simulink model "HelicopterStateEstimation"  (R2023a)
settings: Solver=ode4  StartTime=0.0  StopTime=15  FixedStep=0.1  RelTol=1e-3
values from neighbouring files (symbols this model uses):
  A_c = [0, 0, 1, 0 ... (first row only)    [init.m]
  B_c = [0, 0 ... (first row only)    [init.m]
  B_p = 0.01    [init.m]
  B_y = 0.08    [init.m]
  C_c = [1,0,0,0 ... (first row only)    [init.m]
  g = 9.81    [init.m]
  j_eq_p = 0.0172    [init.m]
  j_eq_y = 0.0210    (= 0.021)    [init.m]
  K_pp = 0.0556    [init.m]
  K_py = 0.005    [init.m]
  K_yp = 0.15    [init.m]
  K_yy = 0.21084    [init.m]
  l_cm = 0.015    [init.m]
  m_heli = 0.479    [init.m]
  psi_op = pi/2    (= 1.57079632679)    [init.m]
  teta_op = -10*pi/180    (= -0.174532925199)    [init.m]
  V_mp_op = K_yy*m_heli*g*cos(teta_op)*l_cm/(K_yy*K_pp - K_yp*K_py)    [init.m]
  v_my_op = K_yp*V_mp_op/K_yy    [init.m]
  wpsi_op = 0    [init.m]
  wteta_op = 0    [init.m]
undefined symbols (not defined in the file or in its folder): L
libraries: simulink_extras x6
settings Model: Creator=Jardar Fagerlund  LastModifiedBy=Jardar Fagerlund

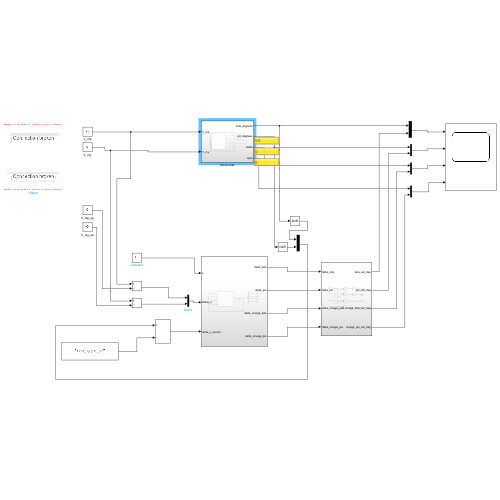
[thumbnail: Simulink's stored preview of the top-level diagram]
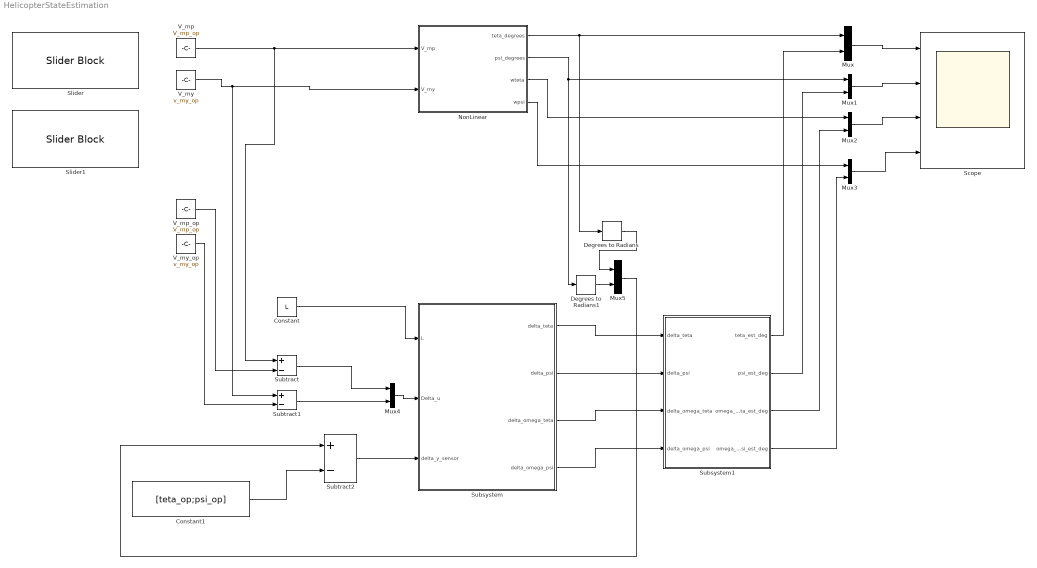
== system HelicopterStateEstimation ==
  Constant : Constant  Value=L
  Constant1 : Constant  Value=[teta_op;psi_op]
  Degrees to Radians : simulink_extras/Transformations/Degrees to Radians
  Degrees to Radians1 : simulink_extras/Transformations/Degrees to Radians
  Mux{,1..5} (6 alike) : Mux  Inputs=2
  NonLinear : Subsystem
  Scope : Scope  NumInputPorts=4
  Slider : SliderBlock  ScaleMin=1.1  ScaleMax=1.23
  Slider1 : SliderBlock  ScaleMin=0.4  ScaleMax=1
  Subsystem : Subsystem
  Subsystem1 : Subsystem
  Subtract : Sum  Inputs=+-
  Subtract1 : Sum  Inputs=+-
  Subtract2 : Sum  Inputs=+-
  V_mp : Constant  Value=V_mp_op
  V_mp_op : Constant  Value=V_mp_op
  V_my : Constant  Value=v_my_op
  V_my_op : Constant  Value=v_my_op
  wires:
  V_mp/1 -> Subtract/1, NonLinear/1(V_mp)
  V_my/1 -> NonLinear/2(V_my), Subtract1/1
  NonLinear/1(teta_degrees) -> Degrees to Radians/1, Mux/1
  NonLinear/2(psi_degrees) -> Degrees to Radians1/1, Mux1/1
  Mux/1 -> Scope/1
  Mux1/1 -> Scope/2
  Mux2/1 -> Scope/3
  Mux3/1 -> Scope/4
  NonLinear/3(wteta) -> Mux2/1
  NonLinear/4(wpsi) -> Mux3/1
  V_my_op/1 -> Subtract1/2
  Constant/1 -> Subsystem/1(L)
  Subtract/1 -> Mux4/1
  Subtract1/1 -> Mux4/2
  Mux4/1 -> Subsystem/2(Delta_u)
  Subtract2/1 -> Subsystem/3(delta_y_sensor)
  Constant1/1 -> Subtract2/2
  Mux5/1 -> Subtract2/1
  V_mp_op/1 -> Subtract/2
  Subsystem/1(delta_teta) -> Subsystem1/1(delta_teta)
  Subsystem/2(delta_psi) -> Subsystem1/2(delta_psi)
  Subsystem/3(delta_omega_teta) -> Subsystem1/3(delta_omega_teta)
  Subsystem/4(delta_omega_psi) -> Subsystem1/4(delta_omega_psi)
  Subsystem1/1(teta_est_deg) -> Mux/2
  Subsystem1/2(psi_est_deg) -> Mux1/2
  Subsystem1/3(omega_teta_est_deg) -> Mux2/2
  Subsystem1/4(omega_psi_est_deg) -> Mux3/2
  Degrees to Radians1/1 -> Mux5/2
  Degrees to Radians/1 -> Mux5/1

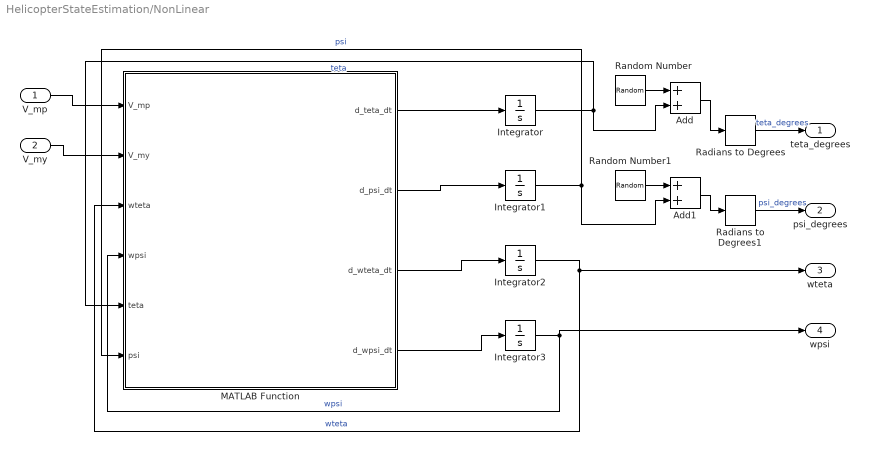
== system HelicopterStateEstimation/NonLinear ==
  V_mp : Inport
  V_my : Inport  Port=2
  Add : Sum
  Add1 : Sum
  Integrator : Integrator  InitialCondition=teta_op  LimitOutput=on  UpperSaturationLimit=35*pi/180  LowerSaturationLimit=-45*pi/180
  Integrator1 : Integrator  InitialCondition=psi_op  LimitOutput=on  UpperSaturationLimit=pi  LowerSaturationLimit=0
  Integrator2 : Integrator  InitialCondition=wteta_op
  Integrator3 : Integrator  InitialCondition=wpsi_op
  MATLAB Function : MATLAB Function  TreatAsAtomicUnit=on
  Radians to Degrees : simulink_extras/Transformations/Radians to Degrees
  Radians to Degrees1 : simulink_extras/Transformations/Radians to Degrees
  Random Number : RandomNumber  Variance=0.01
  Random Number1 : RandomNumber  Variance=0.01
  teta_degrees : Outport
  psi_degrees : Outport  Port=2
  wteta : Outport  Port=3
  wpsi : Outport  Port=4
  wires:
  Integrator/1 -> Add/2, MATLAB Function/5(teta)  "teta"
  MATLAB Function/3(d_wteta_dt) -> Integrator2/1
  MATLAB Function/1(d_teta_dt) -> Integrator/1
  Integrator1/1 -> Add1/2, MATLAB Function/6(psi)  "psi"
  MATLAB Function/4(d_wpsi_dt) -> Integrator3/1
  Integrator2/1 -> wteta/1, MATLAB Function/3(wteta)  "wteta"
  V_mp/1 -> MATLAB Function/1(V_mp)
  MATLAB Function/2(d_psi_dt) -> Integrator1/1
  Integrator3/1 -> wpsi/1, MATLAB Function/4(wpsi)  "wpsi"
  Radians to Degrees/1 -> teta_degrees/1  "teta_degrees"
  Radians to Degrees1/1 -> psi_degrees/1  "psi_degrees"
  V_my/1 -> MATLAB Function/2(V_my)
  Random Number/1 -> Add/1
  Add/1 -> Radians to Degrees/1
  Random Number1/1 -> Add1/1
  Add1/1 -> Radians to Degrees1/1

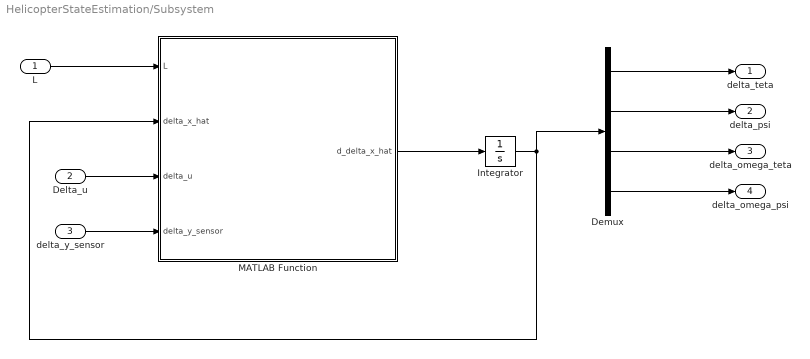
== system HelicopterStateEstimation/Subsystem ==
  L : Inport
  Delta_u : Inport  Port=2
  delta_y_sensor : Inport  Port=3
  Demux : Demux
  Integrator : Integrator  InitialCondition=[-20*pi/180;20*pi/180;0;0];  LimitOutput=on  UpperSaturationLimit=[45*pi/180 - teta_op; pi-psi_op;inf;inf];  LowerSaturationLimit=[-45*pi/180-teta_op; 0-psi_op; -inf;-inf];
  MATLAB Function : MATLAB Function  TreatAsAtomicUnit=on
  delta_teta : Outport
  delta_psi : Outport  Port=2
  delta_omega_teta : Outport  Port=3
  delta_omega_psi : Outport  Port=4
  wires:
  L/1 -> MATLAB Function/1(L)
  MATLAB Function/1(d_delta_x_hat) -> Integrator/1
  Integrator/1 -> MATLAB Function/2(delta_x_hat), Demux/1
  Delta_u/1 -> MATLAB Function/3(delta_u)
  delta_y_sensor/1 -> MATLAB Function/4(delta_y_sensor)
  Demux/4 -> delta_omega_psi/1
  Demux/3 -> delta_omega_teta/1
  Demux/2 -> delta_psi/1
  Demux/1 -> delta_teta/1

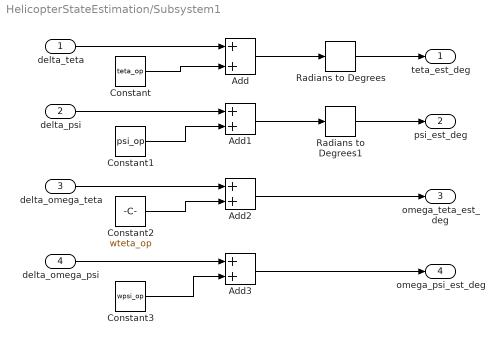
== system HelicopterStateEstimation/Subsystem1 ==
  delta_teta : Inport
  delta_psi : Inport  Port=2
  delta_omega_teta : Inport  Port=3
  delta_omega_psi : Inport  Port=4
  Add{,1..3} (4 alike) : Sum
  Constant : Constant  Value=teta_op
  Constant1 : Constant  Value=psi_op
  Constant2 : Constant  Value=wteta_op
  Constant3 : Constant  Value=wpsi_op
  Radians to Degrees : simulink_extras/Transformations/Radians to Degrees
  Radians to Degrees1 : simulink_extras/Transformations/Radians to Degrees
  teta_est_deg : Outport
  psi_est_deg : Outport  Port=2
  omega_teta_est_deg : Outport  Port=3
  omega_psi_est_deg : Outport  Port=4
  wires:
  Add1/1 -> Radians to Degrees1/1
  Add/1 -> Radians to Degrees/1
  delta_teta/1 -> Add/1
  delta_omega_psi/1 -> Add3/1
  delta_omega_teta/1 -> Add2/1
  delta_psi/1 -> Add1/1
  Constant/1 -> Add/2
  Constant1/1 -> Add1/2
  Constant2/1 -> Add2/2
  Constant3/1 -> Add3/2
  Radians to Degrees/1 -> teta_est_deg/1
  Radians to Degrees1/1 -> psi_est_deg/1
  Add3/1 -> omega_psi_est_deg/1
  Add2/1 -> omega_teta_est_deg/1

== matlab function HelicopterStateEstimation/NonLinear/MATLAB Function ==
  data: V_mp input; d_teta_dt output; V_my input; wteta input; wpsi input; teta input; psi input; d_psi_dt output; d_wteta_dt output; d_wpsi_dt output; K_pp parameter; K_yy parameter; l_cm parameter; m_heli parameter; j_eq_p parameter; j_eq_y parameter; g parameter; K_py parameter; K_yp parameter; B_p parameter; B_y parameter
function [d_teta_dt, d_psi_dt, d_wteta_dt, d_wpsi_dt] = HelicopterSimNonLinear(V_mp, V_my, wteta, wpsi, teta, psi, K_pp,K_yy,l_cm, m_heli, j_eq_p, j_eq_y, g, K_py, K_yp, B_p, B_y)

d_teta_dt = wteta;
d_psi_dt = wpsi;
d_wteta_dt = K_pp*V_mp/(j_eq_p + m_heli*l_cm^2) - K_py*V_my/(j_eq_p + m_heli*l_cm^2) - (B_p*wteta + m_heli*wpsi^2*sin(teta)*l_cm^2*cos(teta)+ m_heli*g*cos(teta)*l_cm)/(j_eq_p + m_heli*l_cm^2);
d_wpsi_dt = K_yp*V_mp/(j_eq_y + m_heli*cos(teta)^2*l_cm^2) - K_yy*V_my/(j_eq_y + m_heli*cos(teta)^2*l_cm^2) + 2*m_heli*wpsi*sin(teta)*l_cm^2*cos(teta)*wteta/(j_eq_y + m_heli*cos(teta)^2*l_cm^2) - B_y*wpsi/(j_eq_y+m_heli*cos(teta)^2*l_cm^2);

== matlab function HelicopterStateEstimation/Subsystem/MATLAB Function ==
  data: L input; d_delta_x_hat output; delta_x_hat input; delta_u input; delta_y_sensor input; A_c parameter; B_c parameter; C_c parameter
function d_delta_x_hat = StateEstimation(L, delta_x_hat, delta_u, delta_y_sensor, A_c, B_c, C_c)

d_delta_x_hat = A_c*delta_x_hat + B_c*delta_u + L*(delta_y_sensor - C_c*delta_x_hat);
